simulink model "Elicottero_fuori_master"  (R2026a)
settings: Solver=ode45  StopTime=20.0
values from neighbouring files (symbols this model uses):
  Acc_Period = fmax / f_Acceler    [Params_Progetto_master.m]
  c_alpha = 0.01    [Params_Progetto.m]    (also in Params_Progetto_master.m; parameters.m; parameters_parametrico.m)
  c_beta = 0.01    [Params_Progetto.m]    (also in Params_Progetto_master.m; parameters.m; parameters_parametrico.m)
  dt = 1/90    (= 0.0111111111111)    [Params_Progetto.m]    (also in Params_Progetto_master.m = 1 / fmax; metriche.m = median(diff(t)))
  eps_p = 0.1    [Params_Progetto.m]    (also in Params_Progetto_master.m; parameters.m; parameters_parametrico.m)
  eps_y = 0.1    [Params_Progetto.m]    (also in Params_Progetto_master.m; parameters.m; parameters_parametrico.m)
  g = 9.81    [Params_Progetto.m]    (also in Params_Progetto_master.m; parameters.m; parameters_parametrico.m)
  h0 = 0.30    (= 0.3)    [Params_Progetto.m]
  I_b = 0.00023    [Params_Progetto.m]    (also in Params_Progetto_master.m; parameters.m; parameters_parametrico.m)
  J_alpha = 0.012    [Params_Progetto.m]    (also in Params_Progetto_master.m; parameters.m; parameters_parametrico.m)
  J_y = 0.00023    [Params_Progetto.m]    (also in Params_Progetto_master.m; parameters.m; parameters_parametrico.m)
  J_z = 0.00364    [Params_Progetto.m]    (also in Params_Progetto_master.m; parameters.m; parameters_parametrico.m)
  l = 0.2    [Params_Progetto.m]    (also in Params_Progetto_master.m; parameters.m; parameters_parametrico.m)
  m = 0.2    [Params_Progetto.m]    (also in Params_Progetto_master.m; parameters.m; parameters_parametrico.m)
  P0_EKF = diag([ ... (first row only)    [Params_Progetto.m]    (also in Params_Progetto_master.m; parameters.m = diag([1, 1, 1, 1]); parameters_parametrico.m = diag([10, 10, 10, 10]))
  Q_EKF = diag([ ... (first row only)    [Params_Progetto.m]    (also in Params_Progetto_master.m; parameters.m = diag([1e-6, 1e-4, 1e-6, 1e-4]); parameters_parametrico.m = diag([1e-5, 1e-3, 1e-5, 1e-3]))
  Q_process = diag([sigma_alpha^2, sigma_beta^2, sigma_d_alpha^2, sigma_d_beta^2])    [Params_Progetto.m]    (also in Params_Progetto_master.m)
  R_EKF = diag([ ... (first row only)    [Params_Progetto.m]    (also in Params_Progetto_master.m; parameters.m = diag([std_dev_cam^2, std_dev_cam^2, std_dev_acc^2]); parameters_parametrico.m)
  R_sens = [sigma_alpha_sensor^2       0                    0;                  0          sigma_cam_sensor^2          0;                  0                0                 sigma_cam_sensor^2]    [Params_Progetto.m]    (also in Params_Progetto_master.m = [sigma_cam_sensor^2       0                    0;           )
  sigma_acc_sensor = 0.05    [Params_Progetto.m]    (also in Params_Progetto_master.m)
  sigma_alpha_sensor = 0.01    [Params_Progetto.m]
  sigma_cam_sensor = 0.002    [Params_Progetto.m]    (also in Params_Progetto_master.m = 0.005)
  Ts_Acceler = 1 / 80    (= 0.0125)    [Params_Progetto.m]    (also in Params_Progetto_master.m)
  Ts_EKF = 1/104    (= 0.00961538461538)    [Params_Progetto.m]    (also in Params_Progetto_master.m)
  Ts_ToF_alpha = 1 / 30    (= 0.0333333333333)    [Params_Progetto.m]
  Ts_Tof_cam = 1/45    (= 0.0222222222222)    [Params_Progetto.m]    (also in Params_Progetto_master.m = 0.00833333333333)
  W0 = ones(1, N)/N    [Params_Progetto.m]    (also in Params_Progetto_master.m)
  X0 = zeros(4, N)    [Params_Progetto.m]    (also in Params_Progetto_master.m)
  x0_EKF = [0; 0; 0; 0]    [Params_Progetto.m]    (also in Params_Progetto_master.m; parameters.m; parameters_parametrico.m = [pi/2; 0.2; pi/4; -0.15])
  XY_Period = fmax / f_cam    [Params_Progetto_master.m]
libraries: simulink x3
settings Model: PacingRate=100  Creator=filin  LastModifiedBy=filin

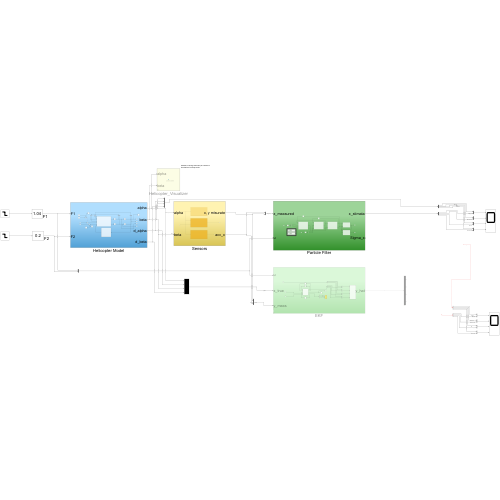
[thumbnail: Simulink's stored preview of the top-level diagram]
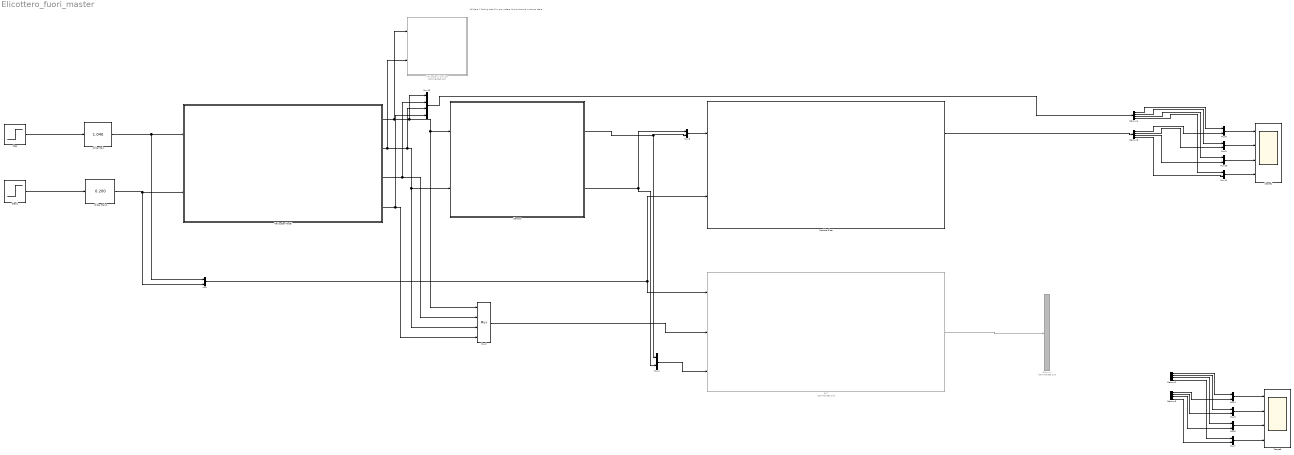
== system Elicottero_fuori_master ==
  note: Abilitare il Pacing sotto Run per vedere la simulazione in tempo reale
  Demux1 : Demux  Commented=on
  Demux{2..5} (4 alike) : Demux
  EKF : Subsystem  Commented=on
  Helicopter Model : Subsystem
  Helicopter_Visualizer : MATLAB Function  Commented=on  TreatAsAtomicUnit=on
  Mux{,1,3..11} (11 alike) : Mux  Inputs=2
  Mux12 : Mux
  Mux2 : Mux
  Particle Filter : Subsystem
  Scope1 : Scope  NumInputPorts=4
      settings: ActiveDisplayYMinimum=-0.45471191819526924  ActiveDisplayYMaximum=1.1125485419212897  DataLoggingVariableName=ScopeData7
  Scope6 : Scope  NumInputPorts=4
      settings: ActiveDisplayYMinimum=-0.15201158861143643  ActiveDisplayYMaximum=0.38619052418530353  DataLoggingVariableName=ScopeData8
  Sensors : Subsystem
  Slider Gain : simulink/Math Operations/Slider Gain  gain=1.040  low=0  high=4
  Slider Gain1 : simulink/Math Operations/Slider Gain  gain=0.200  low=-1  high=1
  Step : Step  InitialValue=1  FinalValue=0  SampleTime=0
  Step1 : Step  InitialValue=1  FinalValue=0  SampleTime=0
  wires:
  Step1/1 -> Slider Gain1/1
  Slider Gain1/1 -> Helicopter Model/2(F2), Mux/2  "F2"
  Step/1 -> Slider Gain/1
  Slider Gain/1 -> Helicopter Model/1(F1), Mux/1  "F1"
  Helicopter Model/1(alpha) -> Helicopter_Visualizer/1(alpha), Mux12/1, Mux2/1, Sensors/1(alpha)  "alpha"
  Helicopter Model/2(beta) -> Mux12/3, Mux2/3, Sensors/2(beta), Helicopter_Visualizer/2(beta)  "beta"
  Mux/1 -> EKF/1(u), Particle Filter/2(In1)
  EKF/1(y_hat) -> Demux1/1
  Sensors/2(h_misurato_diagonale) -> Mux1/2, Mux3/1  "acc_mis"
  Mux1/1 -> EKF/3(y_meas)  "y_meas"
  Demux3/2 -> Mux5/2  "alpha_dot_hat"
  Demux3/4 -> Mux7/2  "beta_dot_hat"
  Demux2/4 -> Mux7/1  "beta_dot"
  Demux3/3 -> Mux6/2  "beta_hat"
  Demux3/1 -> Mux4/2  "alpha_hat"
  Mux4/1 -> Scope6/1
  Mux7/1 -> Scope6/4
  Mux6/1 -> Scope6/3
  ? -> Demux3/1
  Demux2/2 -> Mux5/1  "alpha_dot"
  Demux2/3 -> Mux6/1  "beta"
  Mux5/1 -> Scope6/2
  ? -> Demux2/1  "x_true"
  Demux2/1 -> Mux4/1  "alpha"
  Helicopter Model/4(Out4) -> Mux12/4, Mux2/4
  Helicopter Model/3(Out3) -> Mux12/2, Mux2/2
  Mux2/1 -> EKF/2(x_true)  "x_true"
  Sensors/1(z_measured1) -> Mux3/2, Mux1/1
  Mux3/1 -> Particle Filter/1(z_measured)  "acc_x, x, y"
  Demux5/3 -> Mux10/2  "beta_hat"
  Demux5/4 -> Mux11/2  "beta_dot_hat"
  Mux11/1 -> Scope1/4
  Demux4/2 -> Mux9/1  "alpha_dot"
  Mux9/1 -> Scope1/2
  Demux5/1 -> Mux8/2  "alpha_hat"
  Demux4/4 -> Mux11/1  "beta_dot"
  Demux4/1 -> Mux8/1  "alpha"
  Mux8/1 -> Scope1/1
  Demux4/3 -> Mux10/1  "beta"
  Mux10/1 -> Scope1/3
  Demux5/2 -> Mux9/2  "alpha_dot_hat"
  Particle Filter/1(x_stimata) -> Demux5/1
  Mux12/1 -> Demux4/1

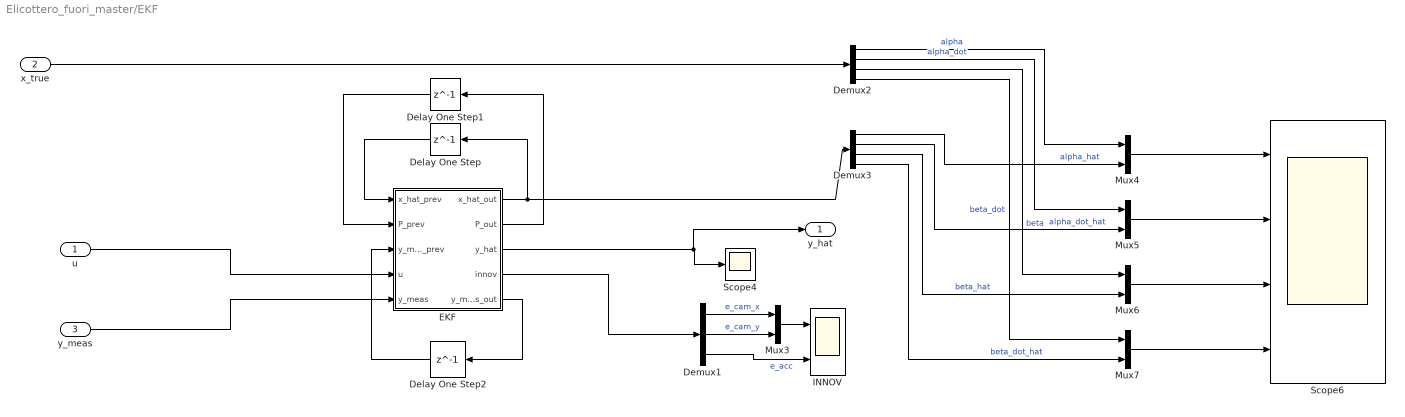
== system Elicottero_fuori_master/EKF ==
  u : Inport
  x_true : Inport  Port=2
  y_meas : Inport  Port=3
  Delay One Step : Delay  DelayLength=1  InitialCondition=x0_EKF  SampleTime=Ts_EKF
  Delay One Step1 : Delay  DelayLength=1  InitialCondition=P0_EKF  SampleTime=Ts_EKF
  Delay One Step2 : Delay  DelayLength=1  InitialCondition=[NaN; NaN; NaN]  SampleTime=Ts_EKF
  Demux1 : Demux  Outputs=3
  Demux2 : Demux
  Demux3 : Demux
  EKF : MATLAB Function  TreatAsAtomicUnit=on
  INNOV : Scope  NumInputPorts=2
      settings: ActiveDisplayYMinimum=-0.3095222726875051  ActiveDisplayYMaximum=0.43177739426795658  DataLoggingVariableName=ScopeData6
  Mux{3..7} (5 alike) : Mux  Inputs=2
  Scope4 : Scope
      settings: ActiveDisplayYMinimum=-0.80524166083087523  ActiveDisplayYMaximum=1.1715327148927259  DataLoggingVariableName=ScopeData5
  Scope6 : Scope  NumInputPorts=4
      settings: ActiveDisplayYMinimum=-0.26940186630110513  ActiveDisplayYMaximum=0.82794320070456306
  y_hat : Outport
  wires:
  EKF/5(y_meas_out) -> Delay One Step2/1
  Delay One Step2/1 -> EKF/3(y_meas_prev)
  Delay One Step1/1 -> EKF/2(P_prev)
  Delay One Step/1 -> EKF/1(x_hat_prev)
  EKF/2(P_out) -> Delay One Step1/1
  EKF/3(y_hat) -> y_hat/1, Scope4/1
  y_meas/1 -> EKF/5(y_meas)
  u/1 -> EKF/4(u)
  Demux1/2 -> Mux3/2  "e_cam_y"
  EKF/4(innov) -> Demux1/1
  Demux1/1 -> Mux3/1  "e_cam_x"
  Mux3/1 -> INNOV/1
  Demux1/3 -> INNOV/2  "e_acc"
  Demux3/2 -> Mux5/2  "alpha_dot_hat"
  Demux3/4 -> Mux7/2  "beta_dot_hat"
  Demux2/4 -> Mux7/1  "beta_dot"
  Demux3/3 -> Mux6/2  "beta_hat"
  Demux3/1 -> Mux4/2  "alpha_hat"
  Mux4/1 -> Scope6/1
  Mux7/1 -> Scope6/4
  Mux6/1 -> Scope6/3
  EKF/1(x_hat_out) -> Delay One Step/1, Demux3/1
  Demux2/2 -> Mux5/1  "alpha_dot"
  Demux2/3 -> Mux6/1  "beta"
  Mux5/1 -> Scope6/2
  Demux2/1 -> Mux4/1  "alpha"
  x_true/1 -> Demux2/1

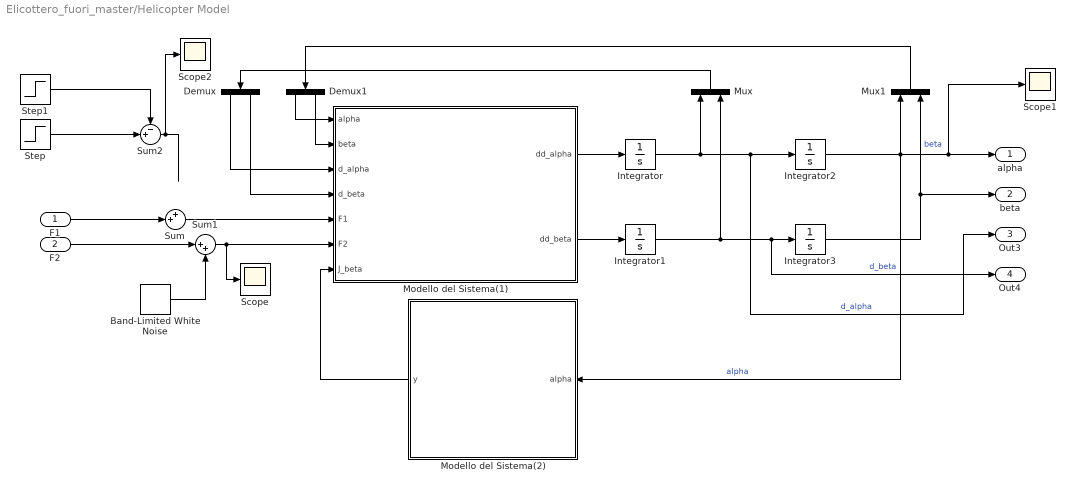
== system Elicottero_fuori_master/Helicopter Model ==
  F1 : Inport
  F2 : Inport  Port=2
  Band-Limited White Noise : simulink/Sources/Band-Limited White Noise  Cov=[0.03]  Ts=0.1  seed=[13541]
  Demux : Demux  Outputs=2
  Demux1 : Demux  Outputs=2
  Integrator : Integrator
  Integrator1 : Integrator
  Integrator2 : Integrator
  Integrator3 : Integrator  WrapState=on
  Modello del Sistema(1) : MATLAB Function  TreatAsAtomicUnit=on
  Modello del Sistema(2) : MATLAB Function  TreatAsAtomicUnit=on
  Mux : Mux  Inputs=2
  Mux1 : Mux  Inputs=2
  Scope : Scope
      settings: ActiveDisplayYMinimum=-5.4959087055113871  ActiveDisplayYMaximum=6.6038183937318049
  Scope1 : Scope
      settings: ActiveDisplayYMinimum=-3.2676033452481468  ActiveDisplayYMaximum=2.2716078537246789  DataLoggingVariableName=ScopeData2
  Scope2 : Scope
      settings: ActiveDisplayYMinimum=-0.73599319291010956  ActiveDisplayYMaximum=2.4547107133398915  DataLoggingVariableName=ScopeData3
  Step : Step  Time=14  FinalValue=5  SampleTime=0
  Step1 : Step  Time=14.1  FinalValue=5  SampleTime=0
  Sum : Sum  Inputs=++|
  Sum1 : Sum  Inputs=|++
  Sum2 : Sum  Inputs=-+|
  alpha : Outport
  beta : Outport  Port=2
  Out3 : Outport  Port=3
  Out4 : Outport  Port=4
  wires:
  Demux1/2 -> Modello del Sistema(1)/2(beta)
  Integrator1/1 -> Mux/2, Out4/1, Integrator3/1  "d_beta"
  Mux/1 -> Demux/1
  Demux/2 -> Modello del Sistema(1)/4(d_beta)
  Modello del Sistema(2)/1(y) -> Modello del Sistema(1)/7(J_beta)
  Demux/1 -> Modello del Sistema(1)/3(d_alpha)
  Integrator3/1 -> beta/1, Mux1/2  "beta"
  Modello del Sistema(1)/1(dd_alpha) -> Integrator/1
  Modello del Sistema(1)/2(dd_beta) -> Integrator1/1
  Demux1/1 -> Modello del Sistema(1)/1(alpha)
  Integrator/1 -> Mux/1, Out3/1, Integrator2/1  "d_alpha"
  Mux1/1 -> Demux1/1
  F1/1 -> Sum/2
  Sum/1 -> Modello del Sistema(1)/5(F1)
  F2/1 -> Sum1/1
  Band-Limited White Noise/1 -> Sum1/2
  Sum1/1 -> Scope/1, Modello del Sistema(1)/6(F2)
  Step/1 -> Sum2/2
  Sum2/1 -> Scope2/1
  Step1/1 -> Sum2/1
  Integrator2/1 -> Modello del Sistema(2)/1(alpha), Mux1/1, Scope1/1, alpha/1  "alpha"

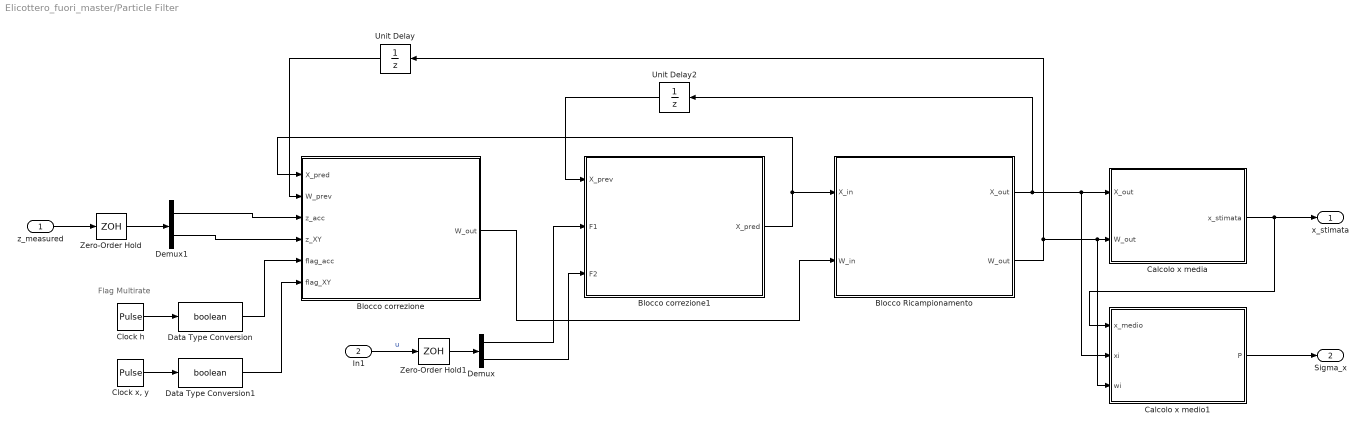
== system Elicottero_fuori_master/Particle Filter ==
  note: Flag Multirate
  z_measured : Inport
  In1 : Inport  Port=2
  Blocco Ricampionamento : MATLAB Function  TreatAsAtomicUnit=on
  Blocco correzione : MATLAB Function  TreatAsAtomicUnit=on
  Blocco correzione1 : MATLAB Function  TreatAsAtomicUnit=on
  Calcolo x media : MATLAB Function  TreatAsAtomicUnit=on
  Calcolo x medio1 : MATLAB Function  TreatAsAtomicUnit=on
  Clock h : DiscretePulseGenerator  Period=Acc_Period  SampleTime=dt
  "Clock x, y" : DiscretePulseGenerator  Period=XY_Period  SampleTime=dt
  Data Type Conversion : DataTypeConversion  OutDataTypeStr=boolean  SaturateOnIntegerOverflow=off  RndMeth=Floor
  Data Type Conversion1 : DataTypeConversion  OutDataTypeStr=boolean  SaturateOnIntegerOverflow=off  RndMeth=Floor
  Demux : Demux  Outputs=2
  Demux1 : Demux  Outputs=[1, 2]
  Unit Delay : UnitDelay  InitialCondition=W0  SampleTime=dt
  Unit Delay2 : UnitDelay  InitialCondition=X0  SampleTime=dt
  Zero-Order Hold : ZeroOrderHold  SampleTime=dt
  Zero-Order Hold1 : ZeroOrderHold  SampleTime=dt
  x_stimata : Outport
  Sigma_x : Outport  Port=2
  wires:
  Demux/1 -> Blocco correzione1/2(F1)
  Demux/2 -> Blocco correzione1/3(F2)
  Blocco correzione/1(W_out) -> Blocco Ricampionamento/2(W_in)
  Unit Delay/1 -> Blocco correzione/2(W_prev)
  Blocco correzione1/1(X_pred) -> Blocco correzione/1(X_pred), Blocco Ricampionamento/1(X_in)
  Unit Delay2/1 -> Blocco correzione1/1(X_prev)
  Blocco Ricampionamento/1(X_out) -> Unit Delay2/1, Calcolo x medio1/2(xi), Calcolo x media/1(X_out)
  Blocco Ricampionamento/2(W_out) -> Unit Delay/1, Calcolo x medio1/3(wi), Calcolo x media/2(W_out)
  Calcolo x media/1(x_stimata) -> Calcolo x medio1/1(x_medio), x_stimata/1
  "Clock x, y"/1 -> Data Type Conversion1/1
  Clock h/1 -> Data Type Conversion/1
  Data Type Conversion/1 -> Blocco correzione/5(flag_acc)
  Data Type Conversion1/1 -> Blocco correzione/6(flag_XY)
  Demux1/2 -> Blocco correzione/4(z_XY)
  Demux1/1 -> Blocco correzione/3(z_acc)
  z_measured/1 -> Zero-Order Hold/1
  Zero-Order Hold/1 -> Demux1/1
  In1/1 -> Zero-Order Hold1/1  "u"
  Zero-Order Hold1/1 -> Demux/1
  Calcolo x medio1/1(P) -> Sigma_x/1

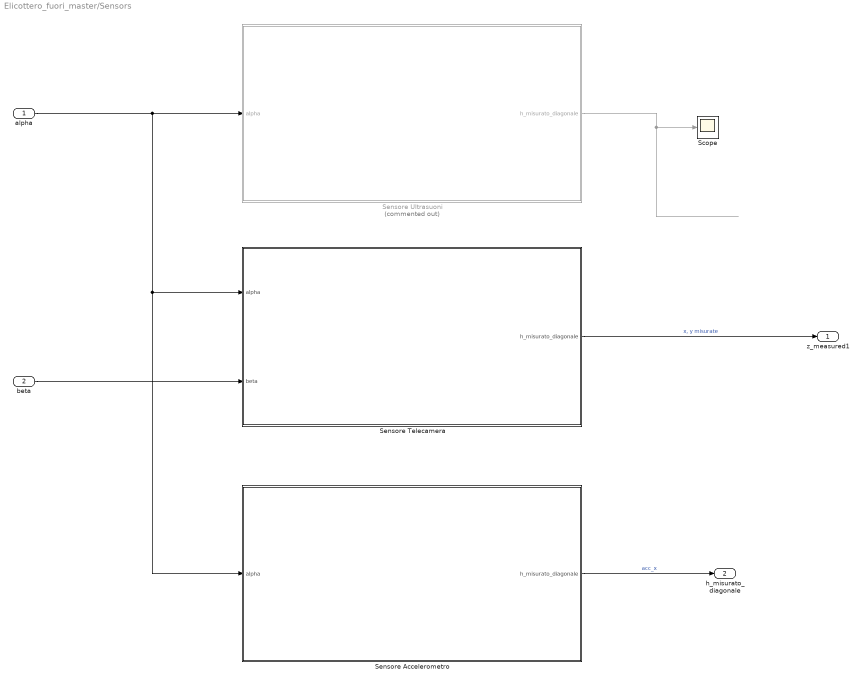
== system Elicottero_fuori_master/Sensors ==
  alpha : Inport
  beta : Inport  Port=2
  Scope : Scope
      settings: ActiveDisplayYMinimum=0.0395682796690905  ActiveDisplayYMaximum=0.56586246991429179  DataLoggingVariableName=ScopeData4
  Sensore Accelerometro : Subsystem
  Sensore Telecamera : Subsystem
  Sensore Ultrasuoni : Subsystem  Commented=on
  z_measured1 : Outport
  h_misurato_diagonale : Outport  Port=2
  wires:
  alpha/1 -> Sensore Accelerometro/1(alpha), Sensore Telecamera/1(alpha), Sensore Ultrasuoni/1(alpha)
  Sensore Ultrasuoni/1(h_misurato_diagonale) -> Scope/1
  Sensore Telecamera/1(h_misurato_diagonale) -> z_measured1/1  "x, y misurate"
  beta/1 -> Sensore Telecamera/2(beta)
  Sensore Accelerometro/1(h_misurato_diagonale) -> h_misurato_diagonale/1  "acc_x"

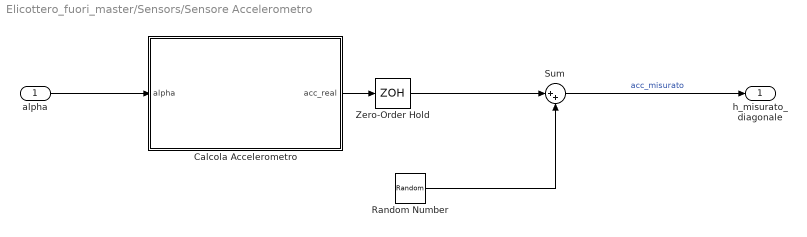
== system Elicottero_fuori_master/Sensors/Sensore Accelerometro ==
  alpha : Inport
  Calcola Accelerometro : MATLAB Function  TreatAsAtomicUnit=on
  Random Number : RandomNumber  Variance=sigma_acc_sensor^2  Seed=1357  SampleTime=Ts_Acceler
  Sum : Sum  Inputs=|++
  Zero-Order Hold : ZeroOrderHold  SampleTime=Ts_Acceler
  h_misurato_diagonale : Outport
  wires:
  Random Number/1 -> Sum/2
  Zero-Order Hold/1 -> Sum/1
  Sum/1 -> h_misurato_diagonale/1  "acc_misurato"
  alpha/1 -> Calcola Accelerometro/1(alpha)
  Calcola Accelerometro/1(acc_real) -> Zero-Order Hold/1

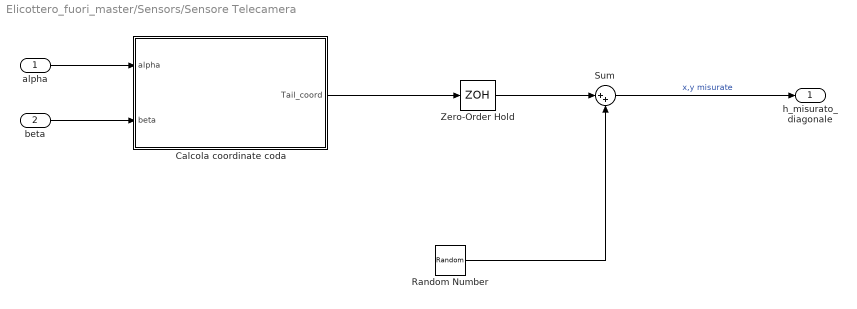
== system Elicottero_fuori_master/Sensors/Sensore Telecamera ==
  alpha : Inport
  beta : Inport  Port=2
  Calcola coordinate coda : MATLAB Function  TreatAsAtomicUnit=on
  Random Number : RandomNumber  Variance=sigma_cam_sensor^2  Seed=1357  SampleTime=Ts_Tof_cam
  Sum : Sum  Inputs=|++
  Zero-Order Hold : ZeroOrderHold  SampleTime=Ts_Tof_cam
  h_misurato_diagonale : Outport
  wires:
  Zero-Order Hold/1 -> Sum/1
  Random Number/1 -> Sum/2
  Sum/1 -> h_misurato_diagonale/1  "x,y misurate"
  Calcola coordinate coda/1(Tail_coord) -> Zero-Order Hold/1
  beta/1 -> Calcola coordinate coda/2(beta)
  alpha/1 -> Calcola coordinate coda/1(alpha)

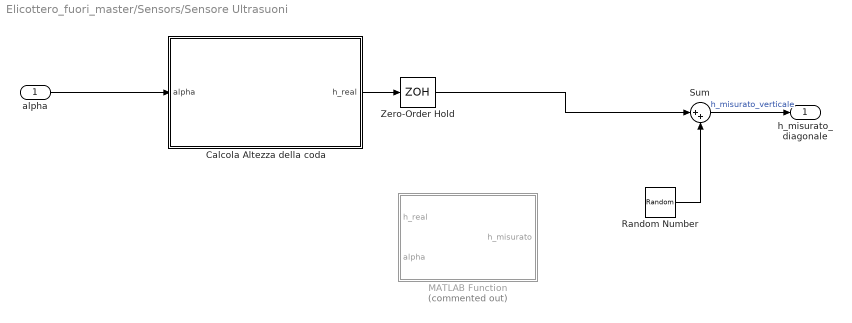
== system Elicottero_fuori_master/Sensors/Sensore Ultrasuoni ==
  alpha : Inport
  Calcola Altezza della coda : MATLAB Function  TreatAsAtomicUnit=on
  MATLAB Function : MATLAB Function  Commented=on  TreatAsAtomicUnit=on
  Random Number : RandomNumber  Variance=sigma_alpha_sensor^2  Seed=1357  SampleTime=Ts_ToF_alpha
  Sum : Sum  Inputs=|++
  Zero-Order Hold : ZeroOrderHold  SampleTime=Ts_ToF_alpha
  h_misurato_diagonale : Outport
  wires:
  Random Number/1 -> Sum/2
  Sum/1 -> h_misurato_diagonale/1  "h_misurato_verticale"
  alpha/1 -> Calcola Altezza della coda/1(alpha)
  Calcola Altezza della coda/1(h_real) -> Zero-Order Hold/1
  Zero-Order Hold/1 -> Sum/1

== matlab function Elicottero_fuori_master/Sensors/Sensore Ultrasuoni/Calcola Altezza della coda ==
  data: alpha input; h_real output; l parameter; h0 parameter
function h_real = Compute_Tail_height(alpha, l, h0)

% Sensore ultrasuoni sotto il muso.
% Misura la distanza verticale del muso dal tavolo.
%
% Modello:
% y_alpha = h0 + l_s_alpha * sin(alpha)

h_real = h0 - l * sin(alpha);

end

== matlab function Elicottero_fuori_master/EKF/EKF ==
  data: x_hat_prev input; P_prev input; y_meas_prev input; u input; x_hat_out output; y_meas input; P_out output; Ts_EKF parameter; Q_EKF parameter; R_EKF parameter; J_alpha parameter; J_y parameter; J_z parameter; I_b parameter; m parameter; l parameter; g parameter; c_alpha parameter; c_beta parameter; eps_p parameter; eps_y parameter; y_hat output; innov output; y_meas_out output
function [x_hat_out, P_out, y_hat, innov, y_meas_out] = EKF_multirate( ...
                                                        x_hat_prev, P_prev, y_meas_prev, u, y_meas, ...
                                                        Ts_EKF, Q_EKF, R_EKF, ...
                                                        J_alpha, J_y, J_z, I_b, m, l, g, ...
                                                        c_alpha, c_beta, eps_p, eps_y)

% EKF multirate per elicottero 2-DOF
%
% Stato:
%   x = [alpha; d_alpha; beta; d_beta]
%
% Ingresso:
%   u = [F1; F2]
%
% Misure:
%   y_meas = [x_cam_mis; y_cam_mis; acc_mis]
%
% Struttura:
%   - predizione sempre a Ts_EKF
%   - correzione camera solo se arriva nuovo campione camera
%   - correzione accelerometro solo se arriva nuovo campione accelerometro
%

% ============================================================
% 0. Rilevamento nuovi campioni sensori
% ============================================================

cam_available = ...
    ((y_meas(1) ~= y_meas_prev(1)) || (y_meas(2) ~= y_meas_prev(2))) ...
    && (~isnan(y_meas(1))) && (~isnan(y_meas(2)));

acc_available = ...
    (y_meas(3) ~= y_meas_prev(3)) ...
    && (~isnan(y_meas(3)));

% salvo la misura corrente per il prossimo passo
y_meas_out = y_meas;

% output debug inizializzati a dimensione fissa
innov = zeros(3,1);

% ============================================================
% 1. Estrazione ingressi
% ============================================================

F1 = u(1);
F2 = u(2);

alpha   = x_hat_prev(1);
d_alpha = x_hat_prev(2);
beta    = x_hat_prev(3);
d_beta  = x_hat_prev(4);

% ============================================================
% 2. Predizione dinamica continua + Eulero
% ============================================================

J_beta = J_y*sin(alpha)^2 + (J_z + m*l^2)*cos(alpha)^2 + I_b;

dd_alpha = ( ...
    - c_alpha*d_alpha ...
    - m*g*l*sin(alpha) ...
    + l*F1*cos(beta) ...
    + eps_p*l*F2*sin(beta) ...
    ) / J_alpha;

dd_beta = ( ...
    - c_beta*d_beta ...
    + l*F2*cos(alpha) ...
    + eps_y*l*F1*sin(alpha) ...
    ) / J_beta;

f = [
    d_alpha;
    dd_alpha;
    d_beta;
    dd_beta
];

x_pred = x_hat_prev + Ts_EKF*f;

% ============================================================
% 3. Jacobiana dinamica A_c e F_k
% ============================================================

Kgeom = J_z + m*l^2;

dJbeta_dalpha = 2*sin(alpha)*cos(alpha)*(J_y - Kgeom);

% Derivate dd_alpha
d_ddalpha_d_alpha = -m*g*l*cos(alpha) / J_alpha;
d_ddalpha_d_dalpha = -c_alpha / J_alpha;

d_ddalpha_d_beta = ( ...
    -l*F1*sin(beta) ...
    + eps_p*l*F2*cos(beta) ...
    ) / J_alpha;

d_ddalpha_d_dbeta = 0;

% Derivate dd_beta
N_beta = ...
    - c_beta*d_beta ...
    + l*F2*cos(alpha) ...
    + eps_y*l*F1*sin(alpha);

dNbeta_dalpha = ...
    - l*F2*sin(alpha) ...
    + eps_y*l*F1*cos(alpha);

d_ddbeta_d_alpha = ...
    (dNbeta_dalpha*J_beta - N_beta*dJbeta_dalpha) / (J_beta^2);

d_ddbeta_d_dalpha = 0;
d_ddbeta_d_beta = 0;
d_ddbeta_d_dbeta = -c_beta / J_beta;

A_c = [
    0,                 1,                  0,                0;
    d_ddalpha_d_alpha, d_ddalpha_d_dalpha, d_ddalpha_d_beta, d_ddalpha_d_dbeta;
    0,                 0,                  0,                1;
    d_ddbeta_d_alpha,  d_ddbeta_d_dalpha,  d_ddbeta_d_beta,  d_ddbeta_d_dbeta
];

F_k = eye(4) + Ts_EKF*A_c;

P_pred = F_k*P_prev*F_k' + Q_EKF;
P_pred = (P_pred + P_pred')/2;

% Dopo la predizione, questi sono gli stati correnti del filtro
x_hat = x_pred;
P = P_pred;

% ============================================================
% 4. Correzione multirate con camera
% ============================================================

if cam_available

    a = x_hat(1);
    b = x_hat(3);

    h_cam = [
        l*cos(a)*cos(b);
        l*cos(a)*sin(b)
    ];

    H_cam = [
        -l*sin(a)*cos(b), 0, -l*cos(a)*sin(b), 0;
        -l*sin(a)*sin(b), 0,  l*cos(a)*cos(b), 0
    ];

    y_cam = y_meas(1:2);
    R_cam = R_EKF(1:2,1:2);

    e_cam = y_cam - h_cam;

    S_cam = H_cam*P*H_cam' + R_cam;

    L_cam = P*H_cam'/S_cam;

    x_hat = x_hat + L_cam*e_cam;

    % Aggiornamento covarianza come a lezione
    P = P - L_cam*S_cam*L_cam';

    %% Simmetrizzazione numerica: 
    % applico una simmetrizzazione numerica;
    % non modifica la struttura del filtro, 
    % mi serve a compensare piccole asimmetrie dovute agli errori di arrotondamento 
    % in virgola mobile 
    %P = (P + P')/2;

    % debug
    innov(1:2) = e_cam;

end

% ============================================================
% 5. Correzione multirate con accelerometro
% ============================================================

if acc_available

    a = x_hat(1);

    h_acc = g*sin(a);

    H_acc = [
        g*cos(a), 0, 0, 0
    ];

    y_acc = y_meas(3);
    R_acc = R_EKF(3,3);

    e_acc = y_acc - h_acc;

    S_acc = H_acc*P*H_acc' + R_acc;

    L_acc = P*H_acc'/S_acc;

    x_hat = x_hat + L_acc*e_acc;

    % Aggiornamento covarianza come a lezione
    P = P - L_acc*S_acc*L_acc';

    %% Simmetrizzazione numerica: 
    % applico una simmetrizzazione numerica;
    % non modifica la struttura del filtro, 
    % mi serve a compensare piccole asimmetrie dovute agli errori di arrotondamento 
    % in virgola mobile 

    %P = (P + P')/2;

    % debug
    innov(3) = e_acc;

end

% ============================================================
% 6. Output finali
% ============================================================

% WRAP degli angoli stimati in [-pi, pi]
x_hat(1) = atan2(sin(x_hat(1)), cos(x_hat(1)));  % alpha
x_hat(3) = atan2(sin(x_hat(3)), cos(x_hat(3)));  % beta

x_hat_out = x_hat;
P_out = P;

% misura stimata finale, utile per scope/debug
a_final = x_hat_out(1);
b_final = x_hat_out(3);

y_hat = [
    l*cos(a_final)*cos(b_final);
    l*cos(a_final)*sin(b_final);
    g*sin(a_final)
];

end

== matlab function Elicottero_fuori_master/Sensors/Sensore Telecamera/Calcola coordinate coda ==
  data: alpha input; beta input; Tail_coord output; l parameter
function Tail_coord = Compute_Tail_coordinates(alpha, beta, l)

x = l * cos(alpha) * cos(beta);
y = l * cos(alpha) * sin(beta);

Tail_coord = [x ; y]; 

end

== matlab function Elicottero_fuori_master/Particle Filter/Blocco correzione ==
  data: X_pred input; W_out output size=[1 N]; W_prev input size=[1 N]; z_acc input; z_XY input; flag_acc input; flag_XY input; l parameter; R_sens parameter; g parameter
function W_out = particle_filter_correction_multirate(X_pred, W_prev, z_acc, z_XY, flag_acc, flag_XY, l, R_sens, g)
    % INGRESSI:
    % X_pred: Matrice [4 x N] particelle
    % W_prev: Vettore [1 x N] pesi
    % z_acc: Scalare (misura diagonale dell'altezza da ultrasuoni)
    % z_XY: Vettore [2 x 1] (misura X, Y della telecamera)
    % flag_L: Booleano (1 se z_acc è un nuovo campione a 30Hz)
    % flag_XY: Booleano (1 se z_XY è un nuovo campione a 45Hz)
    % l, h0: Costanti geometriche dal workspace
    % R_sens: Matrice di covarianza [3 x 3] dal workspace
    
    N = length(W_prev);
    W_out = zeros(1, N); 
    
    % Estrazione delle varianze dalla matrice R_sens [3x3]
    
    inv_R_XY = inv(R_sens(1:2, 1:2));   % Inversa della covarianza telecamera (X-Y)
    var_acc = R_sens(3, 3);             % Varianza dell'accelerometro
    
    for i = 1:N
        alpha_i = X_pred(1, i);
        beta_i  = X_pred(3, i);
        
        % Inizializzo le likelihood a 1 (neutre se il sensore non ha campionato)
        likelihood_acc = 1;
        likelihood_XY = 1;
        
        % --- AGGIORNAMENTO SENSORE accelerazione ---
        if flag_acc == true
            % Calcolo l'altezza teorica
            acc_x_hat = g * sin(alpha_i);
            
            % Errore e Likelihood
            e_acc = z_acc - acc_x_hat;
            likelihood_acc = exp(-0.5 * (e_acc.^2 / var_acc));
        end
        
        % --- AGGIORNAMENTO SENSORE YAW (Telecamera - 45 Hz) ---
        if flag_XY == true
            X_hat = l * cos(alpha_i) * cos(beta_i);
            Y_hat = l * cos(alpha_i) * sin(beta_i);
            
            e_XY = z_XY - [X_hat; Y_hat];
            likelihood_XY = exp(-0.5 * (e_XY' * inv_R_XY * e_XY));
        end
        
        % Il nuovo peso è il prodotto delle probabilità indipendenti
        W_out(i) = W_prev(i) * likelihood_acc * likelihood_XY;
    end
    
    % --- NORMALIZZAZIONE ---
    sum_W = sum(W_out);
    
    % Sicurezza numerica in caso di Particle Depletion
    if sum_W == 0
        W_out = ones(1, N) / N;
    else
        W_out = W_out / sum_W;
    end
end

== matlab function Elicottero_fuori_master/Particle Filter/Blocco correzione1 ==
  data: X_prev input; X_pred output; F1 input; F2 input; dt parameter; J_y parameter; J_z parameter; m parameter; l parameter; I_b parameter; c_alpha parameter; c_beta parameter; g parameter; eps_p parameter; eps_y parameter; J_alpha parameter; Q_process parameter
function X_pred = particle_filter_prediction(X_prev, F1, F2, dt, J_y, J_z, m, l, I_b, c_alpha, c_beta, g, eps_p, eps_y, J_alpha, Q_process)
    
    N = size(X_prev, 2);
    X_pred = zeros(4, N);
    
    sigmas = sqrt(diag(Q_process));
    noise = sigmas .* randn(4, N);
    

    for i = 1:N
        alpha   = X_prev(1, i);
        d_alpha = X_prev(2, i);
        beta    = X_prev(3, i);
        d_beta  = X_prev(4, i);
        
        % Equazioni di modello

        J_beta   = J_y * (sin(alpha) .^ 2) + (J_z + m * l .^ 2) * (cos(alpha)) .^ 2 + I_b; 
        
        dd_alpha = (- c_alpha * d_alpha - m * g * l * sin(alpha) + l * F1...
                    * cos(beta) + eps_p * l * F2 * sin(beta)) / J_alpha;
                    
        dd_beta  = (- c_beta * d_beta + l * F2 * cos(alpha) + eps_y * l * F1...
                    * sin(alpha)) / J_beta;
        
        alpha_next   = alpha + d_alpha * dt;
        
        beta_next    = beta + d_beta * dt;
        beta_next = wrapToPi(beta_next);

        d_alpha_next = d_alpha + dd_alpha * dt;
        d_beta_next  = d_beta + dd_beta * dt;
        
        X_pred(:, i) = [alpha_next; d_alpha_next; beta_next; d_beta_next];
    end
    
    X_pred = X_pred + noise;
end

== matlab function Elicottero_fuori_master/Particle Filter/Calcolo x media ==
  data: X_out input; x_stimata output size=[4, 1]; W_out input size=[1, N]
function x_stimata = dot_prod(X_out, W_out)
    % INGRESSI:
    % X_out : Matrice delle particelle [4 x N]
    % W_out : Vettore riga dei pesi [1 x N] (deve sommare a 1)
    
    % Assicuriamoci che W_out sia un vettore colonna per il prodotto matriciale
    w = W_out(:); 

    % 1. Media lineare per gli stati non angolari (alpha, d_alpha, d_beta)
    alpha_media   = X_out(1, :) * w;
    d_alpha_media = X_out(2, :) * w;
    d_beta_media  = X_out(4, :) * w;

    % 2. MEDIA CIRCOLARE PESATA per lo YAW (beta, indice 3)
    beta_particelle = X_out(3, :);
    
    % Trasformiamo l'angolo di ogni particella in componenti cartesiane
    sin_beta_pesato = sin(beta_particelle) * w;
    cos_beta_pesato = cos(beta_particelle) * w;
    
    % Ricostruiamo l'angolo medio corretto usando l'arcotangente a 4 quadranti
    beta_media = atan2(sin_beta_pesato, cos_beta_pesato);

    % 3. Ricomponiamo il vettore dello stato stimato (4x1)
    x_stimata = [alpha_media; d_alpha_media; beta_media; d_beta_media];
end

== matlab function Elicottero_fuori_master/Particle Filter/Blocco Ricampionamento ==
  settings: updateMethod=DISCRETE
  data: X_in input size=[4 N]; X_out output size=[4 N]; W_in input size=[1 N]; W_out output size=[1 N]; Resampling_th parameter
function [X_out, W_out] = particle_filter_resampling(X_in, W_in, Resampling_th)
    % INGRESSI:
    % X_in: Matrice [4 x N] delle particelle predette (da particle_filter_prediction)
    % W_in: Vettore [1 x N] dei pesi corretti (da particle_filter_correction)
    
    % USCITE:
    % X_out: Matrice [4 x N] delle particelle ricampionate
    % W_out: Vettore [1 x N] dei pesi resettati
    
    N = length(W_in);
    
    % Pre-allocazione obbligatoria per Simulink Coder
    X_out = zeros(4, N);
    W_out = zeros(1, N);
    indices = zeros(1, N);
    
    % Calcolo il numero di particelle efficaci (N_eff)
    N_eff = 1 / sum(W_in.^2);
    
    % Soglia di ricampionamento (solitamente N/2)
    Soglia = Resampling_th * N;
    
    if N_eff < Soglia
        % --- SYSTEMATIC RESAMPLING ---
        % 1. Calcolo la somma cumulativa dei pesi
        cumsum_W = cumsum(W_in);
        
        % 2. Genero i punti di campionamento equidistanti
        step = 1 / N;
        u1 = rand() * step;
        
        i = 1;
        for j = 1:N
            u_j = u1 + step * (j - 1);
            
            % Scorro la somma cumulativa finché non trovo il "gradino" giusto
            while (u_j > cumsum_W(i)) && (i < N)
                i = i + 1;
            end
            
            indices(j) = i;
        end
        
        % 3. Clono le particelle selezionate
        for k = 1:N
            X_out(:, k) = X_in(:, indices(k));
        end
        
        % 4. Resetto tutti i pesi in modo uniforme
        W_out = ones(1, N) / N;
        
    else
        % Se N_eff è ancora alto, non faccio nulla. 
        % Le particelle e i pesi passano intatti.
        X_out = X_in;
        W_out = W_in;
    end
end

== matlab function Elicottero_fuori_master/Particle Filter/Calcolo x medio1 ==
  data: x_medio input; xi input; P output size=[4, 4]; wi input size=[1, N]
function P = calcola_varianza(x_medio, xi, wi)

    diff = xi - x_medio;
    P = diff * (wi .* diff)';
end

== matlab function Elicottero_fuori_master/Sensors/Sensore Accelerometro/Calcola Accelerometro ==
  data: alpha input; acc_real output; g parameter
function acc_real = Compute_Accelerometer(alpha, g)

%%Si assume un accelerometro monoassiale solidale al corpo,
% orientato in modo da misurare la componente della gravità dovuta al pitch.

acc_real = g * sin(alpha);

%acc_real = -g * sin(alpha); quale usiamo?
end

== matlab function Elicottero_fuori_master/Helicopter Model/Modello del Sistema(2) ==
  data: alpha input; y output; J_y parameter; J_z parameter; m parameter; l parameter; I_b parameter
function y = Aggiorna_J_beta(alpha, J_y, J_z, m, l, I_b)

J_beta = J_y * (sin(alpha) ^ 2) + (J_z + m * l ^ 2) * (cos(alpha)) ^ 2 + I_b; 

y = J_beta;

== matlab function Elicottero_fuori_master/Helicopter Model/Modello del Sistema(1) ==
  data: alpha input; beta input; dd_alpha output; d_alpha input; d_beta input; F1 input; F2 input; J_beta input; dd_beta output; c_alpha parameter; m parameter; g parameter; l parameter; eps_p parameter; J_alpha parameter; c_beta parameter; eps_y parameter
function [dd_alpha, dd_beta] = Helicopter_Helicopter(alpha, beta, d_alpha, d_beta, F1, F2, J_beta, c_alpha, m, g, l, eps_p, J_alpha, c_beta, eps_y)

dd_alpha        = (- c_alpha * d_alpha - m * g * l * sin(alpha) + l * F1...
                    * cos(beta) + eps_p * l * F2 * sin(beta)) / J_alpha;

dd_beta        = (- c_beta * d_beta + l * F2 * cos(alpha) + eps_y * l * F1...
                    * sin(alpha)) / J_beta;

== matlab function Elicottero_fuori_master/Helicopter_Visualizer ==
  data: alpha input; beta input
function Disegna_Elicottero_Realtime(alpha, beta)
    % Definisce i dati come persistenti per non ricreare la finestra a ogni step
    persistent f h_pitch h_yaw l;
    
    if isempty(f)
        l = 0.2; % Lunghezza braccio
        f = figure('Name', 'Simulatore Elicottero 2-DoF');
        
        % Subplot 1: Vista Laterale (Pitch)
        subplot(2,1,1);
        hold on; grid on; axis equal;
        axis([-0.3 0.3 -0.3 0.3]);
        plot([0 0], [-0.3 0], 'k', 'LineWidth', 3); % Perno base
        h_pitch = plot([0 0], [0 0], 'b-o', 'LineWidth', 4, 'MarkerSize', 10);
        title('Vista Laterale - Pitch (\alpha)');
        
        % Subplot 2: Vista dall'Alto (Yaw)
        subplot(2,1,2);
        hold on; grid on; axis equal;
        axis([-0.3 0.3 -0.3 0.3]);
        plot(0, 0, 'k+', 'MarkerSize', 10); % Centro
        h_yaw = plot([0 0], [0 0], 'r-o', 'LineWidth', 4, 'MarkerSize', 10);
        title('Vista dall''Alto - Yaw (\beta)');
    end
    
    % Aggiornamento delle coordinate geometriche
    
    % Pitch: rotazione nel piano verticale X-Z
    % Sfasamento di pi (180 gradi) per posizionare il braccio a sinistra a alpha = 0
    alpha_grafico = alpha + pi; 
    
    x_p = l * cos(alpha_grafico);
    z_p = l * sin(alpha_grafico);
    set(h_pitch, 'XData', [0 x_p], 'YData', [0 z_p]);
        
    % Yaw: rotazione nel piano orizzontale X-Y
    beta_grafico = beta + pi; % Trasla anche lo yaw per coerenza visiva
    x_y = l * cos(beta_grafico);
    y_y = l * sin(beta_grafico);
    set(h_yaw, 'XData', [0 x_y], 'YData', [0 y_y]);
    
    drawnow limitrate; % Forza l'aggiornamento grafico
end

== matlab function Elicottero_fuori_master/Sensors/Sensore Ultrasuoni/MATLAB Function ==
  data: h_misurato output; h_real input; alpha input
function h_misurato =  Wenglor_U1KT001(h_real, alpha)

cos_alpha_safe = max(abs(cos(alpha)), 1e-3);

h_misurato = h_real / cos_alpha_safe;

y = h_misurato;
